simulink model "wlan_mac_dcf_hw"  (Simulink 7.7)
settings: Solver=ode45  StartTime=0.0  StopTime=2e4  RelTol=1e-3
PostLoadFcn:
  | wlan_mac_hw_init
InitFcn:
  | wlan_mac_hw_init
StartFcn:
  | wlan_mac_hw_init
values from neighbouring files (symbols this model uses):
  NB_CNTR_NAV = ceil(log2(MAX_NAV * 160))    [wlan_mac_hw_init.m]
  ticks_per_usec = 10    [wlan_mac_hw_init.m]
undefined symbols (not defined in the file or in its folder): gcbh, xlBlockLoadCallback, xlGetNormalizedPeriod
libraries: xbsIndex_r4 x552, xbsEDKLib_r4 x1
(part 4 of 5)

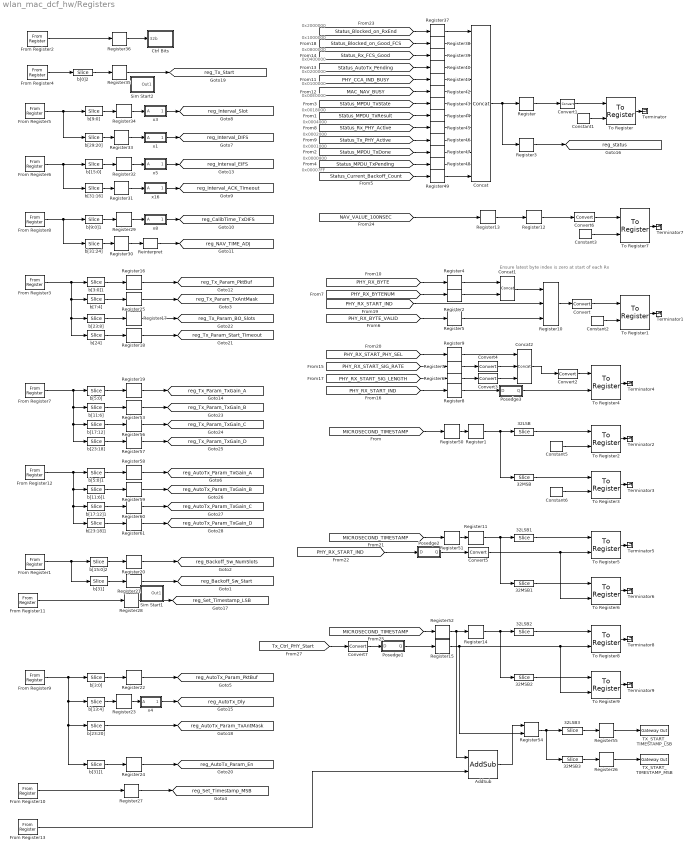
== system wlan_mac_dcf_hw/Registers ==
  note: Ensure latest byte index is zero
      | at start of each Rx
  note: 0x00007FF
  note: 0x0000800
  note: 0x0001000
  note: 0x0002000
  note: 0x0004000
  note: 0x0018000
  note: 0x00E0000
  note: 0x0100000
  note: 0x0200000
  note: 0x0400000
  note: 0x0800000
  note: 0x1000000
  note: 0x2000000
  " b[11:6]" : xbsIndex_r4/Slice  nbits=6  boolean_output=off  mode=Lower Bit Location + Width  bit1=0  base1=MSB of Input  bit0=6  base0=LSB of Input  dbl_ovrd=off  block_type=slice
      settings: block_version=VER_STRING_GOES_HERE
  " b[11:6]1" : xbsIndex_r4/Slice  nbits=6  boolean_output=off  mode=Lower Bit Location + Width  bit1=0  base1=MSB of Input  bit0=6  base0=LSB of Input  dbl_ovrd=off  block_type=slice
      settings: block_version=VER_STRING_GOES_HERE
  " b[13:4]" : xbsIndex_r4/Slice  nbits=10  boolean_output=off  mode=Lower Bit Location + Width  bit1=0  base1=MSB of Input  bit0=4  base0=LSB of Input  dbl_ovrd=off  block_type=slice
      settings: block_version=VER_STRING_GOES_HERE
  " b[15:0]" : xbsIndex_r4/Slice  nbits=16  boolean_output=off  mode=Lower Bit Location + Width  bit1=0  base1=MSB of Input  bit0=0  base0=LSB of Input  dbl_ovrd=off  block_type=slice
      settings: block_version=VER_STRING_GOES_HERE
  " b[15:0]2" : xbsIndex_r4/Slice  nbits=16  boolean_output=off  mode=Lower Bit Location + Width  bit1=0  base1=MSB of Input  bit0=0  base0=LSB of Input  dbl_ovrd=off  block_type=slice
      settings: block_version=VER_STRING_GOES_HERE
  " b[17:12]" : xbsIndex_r4/Slice  nbits=6  boolean_output=off  mode=Lower Bit Location + Width  bit1=0  base1=MSB of Input  bit0=12  base0=LSB of Input  dbl_ovrd=off  block_type=slice
      settings: block_version=VER_STRING_GOES_HERE
  " b[17:12]1" : xbsIndex_r4/Slice  nbits=6  boolean_output=off  mode=Lower Bit Location + Width  bit1=0  base1=MSB of Input  bit0=12  base0=LSB of Input  dbl_ovrd=off  block_type=slice
      settings: block_version=VER_STRING_GOES_HERE
  " b[23:18]" : xbsIndex_r4/Slice  nbits=6  boolean_output=off  mode=Lower Bit Location + Width  bit1=0  base1=MSB of Input  bit0=18  base0=LSB of Input  dbl_ovrd=off  block_type=slice
      settings: block_version=VER_STRING_GOES_HERE
  " b[23:18]1" : xbsIndex_r4/Slice  nbits=6  boolean_output=off  mode=Lower Bit Location + Width  bit1=0  base1=MSB of Input  bit0=18  base0=LSB of Input  dbl_ovrd=off  block_type=slice
      settings: block_version=VER_STRING_GOES_HERE
  " b[23:20]" : xbsIndex_r4/Slice  nbits=4  boolean_output=off  mode=Lower Bit Location + Width  bit1=0  base1=MSB of Input  bit0=20  base0=LSB of Input  dbl_ovrd=off  block_type=slice
      settings: block_version=VER_STRING_GOES_HERE
  " b[23:8]" : xbsIndex_r4/Slice  nbits=16  boolean_output=off  mode=Lower Bit Location + Width  bit1=0  base1=MSB of Input  bit0=8  base0=LSB of Input  dbl_ovrd=off  block_type=slice
      settings: block_version=VER_STRING_GOES_HERE
  " b[24]" : xbsIndex_r4/Slice  nbits=1  boolean_output=on  mode=Lower Bit Location + Width  bit1=0  base1=MSB of Input  bit0=24  base0=LSB of Input  dbl_ovrd=off  block_type=slice
      settings: block_version=VER_STRING_GOES_HERE
  " b[29:20]" : xbsIndex_r4/Slice  nbits=10  boolean_output=off  mode=Lower Bit Location + Width  bit1=0  base1=MSB of Input  bit0=20  base0=LSB of Input  dbl_ovrd=off  block_type=slice
      settings: block_version=VER_STRING_GOES_HERE
  " b[31:16]" : xbsIndex_r4/Slice  nbits=16  boolean_output=off  mode=Lower Bit Location + Width  bit1=0  base1=MSB of Input  bit0=16  base0=LSB of Input  dbl_ovrd=off  block_type=slice
      settings: block_version=VER_STRING_GOES_HERE
  " b[31:24]" : xbsIndex_r4/Slice  nbits=8  boolean_output=off  mode=Lower Bit Location + Width  bit1=0  base1=MSB of Input  bit0=24  base0=LSB of Input  dbl_ovrd=off  block_type=slice
      settings: block_version=VER_STRING_GOES_HERE
  " b[31]" : xbsIndex_r4/Slice  nbits=1  boolean_output=on  mode=Lower Bit Location + Width  bit1=0  base1=MSB of Input  bit0=31  base0=LSB of Input  dbl_ovrd=off  block_type=slice
      settings: block_version=VER_STRING_GOES_HERE
  " b[31]1" : xbsIndex_r4/Slice  nbits=1  boolean_output=on  mode=Lower Bit Location + Width  bit1=0  base1=MSB of Input  bit0=31  base0=LSB of Input  dbl_ovrd=off  block_type=slice
      settings: block_version=VER_STRING_GOES_HERE
  " b[3:0]" : xbsIndex_r4/Slice  nbits=4  boolean_output=off  mode=Lower Bit Location + Width  bit1=0  base1=MSB of Input  bit0=0  base0=LSB of Input  dbl_ovrd=off  block_type=slice
      settings: block_version=VER_STRING_GOES_HERE
  " b[3:0]1" : xbsIndex_r4/Slice  nbits=4  boolean_output=off  mode=Lower Bit Location + Width  bit1=0  base1=MSB of Input  bit0=0  base0=LSB of Input  dbl_ovrd=off  block_type=slice
      settings: block_version=VER_STRING_GOES_HERE
  " b[5:0]" : xbsIndex_r4/Slice  nbits=6  boolean_output=off  mode=Lower Bit Location + Width  bit1=0  base1=MSB of Input  bit0=0  base0=LSB of Input  dbl_ovrd=off  block_type=slice
      settings: block_version=VER_STRING_GOES_HERE
  " b[5:0]1" : xbsIndex_r4/Slice  nbits=6  boolean_output=off  mode=Lower Bit Location + Width  bit1=0  base1=MSB of Input  bit0=0  base0=LSB of Input  dbl_ovrd=off  block_type=slice
      settings: block_version=VER_STRING_GOES_HERE
  " b[7:4]" : xbsIndex_r4/Slice  nbits=4  boolean_output=off  mode=Lower Bit Location + Width  bit1=0  base1=MSB of Input  bit0=4  base0=LSB of Input  dbl_ovrd=off  block_type=slice
      settings: block_version=VER_STRING_GOES_HERE
  " b[9:0]" : xbsIndex_r4/Slice  nbits=10  boolean_output=off  mode=Lower Bit Location + Width  bit1=0  base1=MSB of Input  bit0=0  base0=LSB of Input  dbl_ovrd=off  block_type=slice
      settings: block_version=VER_STRING_GOES_HERE
  " b[9:0]1" : xbsIndex_r4/Slice  nbits=10  boolean_output=off  mode=Lower Bit Location + Width  bit1=0  base1=MSB of Input  bit0=0  base0=LSB of Input  dbl_ovrd=off  block_type=slice
      settings: block_version=VER_STRING_GOES_HERE
  32LSB{,1..3} (4 alike) : xbsIndex_r4/Slice  nbits=32  boolean_output=off  mode=Lower Bit Location + Width  bit1=0  base1=MSB of Input  bit0=0  base0=LSB of Input  dbl_ovrd=off  block_type=slice
      settings: block_version=VER_STRING_GOES_HERE
  32MSB{,1..3} (4 alike) : xbsIndex_r4/Slice  nbits=32  boolean_output=off  mode=Upper Bit Location + Width  bit1=0  base1=MSB of Input  bit0=0  base0=LSB of Input  dbl_ovrd=off  block_type=slice
      settings: block_version=VER_STRING_GOES_HERE
  AddSub : xbsIndex_r4/AddSub  mode=Addition  use_carryin=off  use_carryout=off  en=off  latency=0  precision=User Defined  arith_type=Unsigned  n_bits=64  bin_pt=0  quantization=Truncate  overflow=Wrap  dbl_ovrd=off  use_behavioral_HDL=off  hw_selection=Fabric  pipelined=off  block_type=addsub
  Concat : xbsIndex_r4/Concat  num_inputs=13  dbl_ovrd=off  block_type=concat
      settings: block_version=8.2.02
  Concat1 : xbsIndex_r4/Concat  num_inputs=2  dbl_ovrd=off  block_type=concat
      settings: block_version=8.2.02
  Concat2 : xbsIndex_r4/Concat  num_inputs=3  dbl_ovrd=off  block_type=concat
      settings: block_version=8.2.02
  Constant{1..3,5..6} (5 alike) : xbsIndex_r4/Constant  const=1  gui_display_data_type=Boolean  arith_type=Boolean  n_bits=30  bin_pt=0  preci_type=Single  exp_width=8  frac_width=24  explicit_period=on  period=1  equ=P=C  opselect=C  inp2=PCIN>>17  opr=+  inp1=P  carry=CIN  dbl_ovrd=off  block_type=constant
  Convert{,1..2,6} (4 alike) : xbsIndex_r4/Convert  gui_display_data_type=Fixed-point  arith_type=Unsigned  n_bits=32  bin_pt=0  float_type=Single  exp_bits=8  fraction_bits=24  quantization=Truncate  overflow=Wrap  en=off  latency=0  dbl_ovrd=off  pipeline=off  block_type=convert
  Convert3 : xbsIndex_r4/Convert  gui_display_data_type=Fixed-point  arith_type=Unsigned  n_bits=16  bin_pt=0  float_type=Single  exp_bits=8  fraction_bits=24  quantization=Truncate  overflow=Wrap  en=off  latency=0  dbl_ovrd=off  pipeline=off  block_type=convert
  Convert4 : xbsIndex_r4/Convert  gui_display_data_type=Fixed-point  arith_type=Unsigned  n_bits=8  bin_pt=0  float_type=Single  exp_bits=8  fraction_bits=24  quantization=Truncate  overflow=Wrap  en=off  latency=0  dbl_ovrd=off  pipeline=off  block_type=convert
  Convert5 : xbsIndex_r4/Convert  gui_display_data_type=Boolean  arith_type=Boolean  n_bits=32  bin_pt=0  float_type=Single  exp_bits=8  fraction_bits=24  quantization=Truncate  overflow=Wrap  en=off  latency=0  dbl_ovrd=off  pipeline=off  block_type=convert
  Convert7 : xbsIndex_r4/Convert  gui_display_data_type=Boolean  arith_type=Boolean  n_bits=32  bin_pt=0  float_type=Single  exp_bits=8  fraction_bits=24  quantization=Truncate  overflow=Wrap  en=off  latency=0  dbl_ovrd=off  pipeline=off  block_type=convert
  Ctrl Bits : Subsystem
  From Register1 : xbsIndex_r4/From Register  shared_memory_name='BACKOFF_CTRL'  init=REG_MAC_Backoff_Control  period=1  ownership=Locally owned and initialized  gui_display_data_type=Fixed-point  arith_type=Unsigned  n_bits=32  bin_pt=0  preci_type=Single  dbl_ovrd=off  block_type=fromreg
      settings: AttributesFormatString=<< %<shared_memory_name> >>  infoedit="Register block that reads data to a shared memory register.  Delay of one sample period."
  From Register10 : xbsIndex_r4/From Register  shared_memory_name='TIMESTAMP_SET_MSB'  init=0  period=1  ownership=Locally owned and initialized  gui_display_data_type=Fixed-point  arith_type=Unsigned  n_bits=32  bin_pt=0  preci_type=Single  dbl_ovrd=off  block_type=fromreg
      settings: AttributesFormatString=<< %<shared_memory_name> >>  infoedit="Register block that reads data to a shared memory register.  Delay of one sample period."
  From Register11 : xbsIndex_r4/From Register  shared_memory_name='TIMESTAMP_SET_LSB'  init=0  period=1  ownership=Locally owned and initialized  gui_display_data_type=Fixed-point  arith_type=Unsigned  n_bits=32  bin_pt=0  preci_type=Single  dbl_ovrd=off  block_type=fromreg
      settings: AttributesFormatString=<< %<shared_memory_name> >>  infoedit="Register block that reads data to a shared memory register.  Delay of one sample period."
  From Register12 : xbsIndex_r4/From Register  shared_memory_name='AUTO_TX_GAINS'  init=0  period=1  ownership=Locally owned and initialized  gui_display_data_type=Fixed-point  arith_type=Unsigned  n_bits=32  bin_pt=0  preci_type=Single  dbl_ovrd=off  block_type=fromreg
      settings: AttributesFormatString=<< %<shared_memory_name> >>  infoedit="Register block that reads data to a shared memory register.  Delay of one sample period."
  From Register13 : xbsIndex_r4/From Register  shared_memory_name='TIMESTAMP_INSERT_OFFSET'  init=0  period=1  ownership=Locally owned and initialized  gui_display_data_type=Fixed-point  arith_type="Signed  (2's comp)"  n_bits=32  bin_pt=0  preci_type=Single  dbl_ovrd=off  block_type=fromreg
      settings: AttributesFormatString=<< %<shared_memory_name> >>  infoedit="Register block that reads data to a shared memory register.  Delay of one sample period."
  From Register2 : xbsIndex_r4/From Register  shared_memory_name='Control'  init=REG_MAC_Control  period=1  ownership=Locally owned and initialized  gui_display_data_type=Fixed-point  arith_type=Unsigned  n_bits=32  bin_pt=0  preci_type=Single  dbl_ovrd=off  block_type=fromreg
      settings: AttributesFormatString=<< %<shared_memory_name> >>  infoedit="Register block that reads data to a shared memory register.  Delay of one sample period."
  From Register3 : xbsIndex_r4/From Register  shared_memory_name='MPDU_TX_PARAMS'  init=REG_MAC_MPDU_Tx_Params  period=1  ownership=Locally owned and initialized  gui_display_data_type=Fixed-point  arith_type=Unsigned  n_bits=32  bin_pt=0  preci_type=Single  dbl_ovrd=off  block_type=fromreg
      settings: AttributesFormatString=<< %<shared_memory_name> >>  infoedit="Register block that reads data to a shared memory register.  Delay of one sample period."
  From Register4 : xbsIndex_r4/From Register  shared_memory_name='TX_START'  init=0  period=1  ownership=Locally owned and initialized  gui_display_data_type=Fixed-point  arith_type=Unsigned  n_bits=32  bin_pt=0  preci_type=Single  dbl_ovrd=off  block_type=fromreg
      settings: AttributesFormatString=<< %<shared_memory_name> >>  infoedit="Register block that reads data to a shared memory register.  Delay of one sample period."
  From Register5 : xbsIndex_r4/From Register  shared_memory_name='IFS_INTERVALS1'  init=REG_MAC_Intervals_1  period=1  ownership=Locally owned and initialized  gui_display_data_type=Fixed-point  arith_type=Unsigned  n_bits=32  bin_pt=0  preci_type=Single  dbl_ovrd=off  block_type=fromreg
      settings: AttributesFormatString=<< %<shared_memory_name> >>  infoedit="Register block that reads data to a shared memory register.  Delay of one sample period."
  From Register6 : xbsIndex_r4/From Register  shared_memory_name='IFS_INTERVALS2'  init=REG_MAC_Intervals_2  period=1  ownership=Locally owned and initialized  gui_display_data_type=Fixed-point  arith_type=Unsigned  n_bits=32  bin_pt=0  preci_type=Single  dbl_ovrd=off  block_type=fromreg
      settings: AttributesFormatString=<< %<shared_memory_name> >>  infoedit="Register block that reads data to a shared memory register.  Delay of one sample period."
  From Register7 : xbsIndex_r4/From Register  shared_memory_name='MPDU_TX_GAINS'  init=0  period=1  ownership=Locally owned and initialized  gui_display_data_type=Fixed-point  arith_type=Unsigned  n_bits=32  bin_pt=0  preci_type=Single  dbl_ovrd=off  block_type=fromreg
      settings: AttributesFormatString=<< %<shared_memory_name> >>  infoedit="Register block that reads data to a shared memory register.  Delay of one sample period."
  From Register8 : xbsIndex_r4/From Register  shared_memory_name='CALIB_TIMES'  init=REG_MAC_Calib_Times  period=1  ownership=Locally owned and initialized  gui_display_data_type=Fixed-point  arith_type=Unsigned  n_bits=32  bin_pt=0  preci_type=Single  dbl_ovrd=off  block_type=fromreg
      settings: AttributesFormatString=<< %<shared_memory_name> >>  infoedit="Register block that reads data to a shared memory register.  Delay of one sample period."
  From Register9 : xbsIndex_r4/From Register  shared_memory_name='AUTO_TX_PARAMS'  init=REG_MAC_Auto_Tx_Params  period=1  ownership=Locally owned and initialized  gui_display_data_type=Fixed-point  arith_type=Unsigned  n_bits=32  bin_pt=0  preci_type=Single  dbl_ovrd=off  block_type=fromreg
      settings: AttributesFormatString=<< %<shared_memory_name> >>  infoedit="Register block that reads data to a shared memory register.  Delay of one sample period."
  Posedge1 : Subsystem
  Posedge2 : Subsystem
  Posedge3 : Subsystem
  Register{,1..9,11..53,55..61} (60 alike) : xbsIndex_r4/Register  init=0  rst=off  en=off  dbl_ovrd=off  block_type=register
  Register10 : xbsIndex_r4/Register  init=0  rst=on  en=on  dbl_ovrd=off  block_type=register
  Register54 : xbsIndex_r4/Register  init=0  rst=off  en=on  dbl_ovrd=off  block_type=register
  Reinterpret : xbsIndex_r4/Reinterpret  force_arith_type=on  arith_type="Signed  (2's comp)"  force_bin_pt=off  bin_pt=0  block_type=reinterpret
  Sim Start1 : Subsystem
  Sim Start2 : Subsystem
  TX_START_TIMESTAMP_LSB : xbsIndex_r4/Gateway Out  inherit_from_input=off  hdl_port=on  timing_constraint=None  locs_specified=off  LOCs={}  UseAsDAC=off  DACChannel='1'  block_type=gatewayout
  TX_START_TIMESTAMP_MSB : xbsIndex_r4/Gateway Out  inherit_from_input=off  hdl_port=on  timing_constraint=None  locs_specified=off  LOCs={}  UseAsDAC=off  DACChannel='1'  block_type=gatewayout
  Terminator{,1..9} (10 alike) : Terminator
  To Register : xbsIndex_r4/To Register  shared_memory_name='Status'  init=0  ownership=Locally owned and initialized  explicit_data_type=on  gui_display_data_type=Fixed-point  arith_type=Unsigned  n_bits=32  bin_pt=0  preci_type=Single  dbl_ovrd=off  block_type=toreg
      settings: AttributesFormatString=<< %<shared_memory_name> >>  infoedit="Register block that writes data to a shared memory register.  Delay of one sample period."
  To Register1 : xbsIndex_r4/To Register  shared_memory_name='LATEST_RX_BYTE'  init=0  ownership=Locally owned and initialized  explicit_data_type=on  gui_display_data_type=Fixed-point  arith_type=Unsigned  n_bits=32  bin_pt=0  preci_type=Single  dbl_ovrd=off  block_type=toreg
      settings: AttributesFormatString=<< %<shared_memory_name> >>  infoedit="Register block that writes data to a shared memory register.  Delay of one sample period."
  To Register2 : xbsIndex_r4/To Register  shared_memory_name='TIMESTAMP_LSB'  init=0  ownership=Locally owned and initialized  explicit_data_type=on  gui_display_data_type=Fixed-point  arith_type=Unsigned  n_bits=32  bin_pt=0  preci_type=Single  dbl_ovrd=off  block_type=toreg
      settings: AttributesFormatString=<< %<shared_memory_name> >>  infoedit="Register block that writes data to a shared memory register.  Delay of one sample period."
  To Register3 : xbsIndex_r4/To Register  shared_memory_name='TIMESTAMP_MSB'  init=0  ownership=Locally owned and initialized  explicit_data_type=on  gui_display_data_type=Fixed-point  arith_type=Unsigned  n_bits=32  bin_pt=0  preci_type=Single  dbl_ovrd=off  block_type=toreg
      settings: AttributesFormatString=<< %<shared_memory_name> >>  infoedit="Register block that writes data to a shared memory register.  Delay of one sample period."
  To Register4 : xbsIndex_r4/To Register  shared_memory_name='RX_RATE_LENGTH'  init=0  ownership=Locally owned and initialized  explicit_data_type=on  gui_display_data_type=Fixed-point  arith_type=Unsigned  n_bits=32  bin_pt=0  preci_type=Single  dbl_ovrd=off  block_type=toreg
      settings: AttributesFormatString=<< %<shared_memory_name> >>  infoedit="Register block that writes data to a shared memory register.  Delay of one sample period."
  To Register5 : xbsIndex_r4/To Register  shared_memory_name='RX_START_TIMESTAMP_LSB'  init=0  ownership=Locally owned and initialized  explicit_data_type=on  gui_display_data_type=Fixed-point  arith_type=Unsigned  n_bits=32  bin_pt=0  preci_type=Single  dbl_ovrd=off  block_type=toreg
      settings: AttributesFormatString=<< %<shared_memory_name> >>  infoedit="Register block that writes data to a shared memory register.  Delay of one sample period."
  To Register6 : xbsIndex_r4/To Register  shared_memory_name='RX_START_TIMESTAMP_MSB'  init=0  ownership=Locally owned and initialized  explicit_data_type=on  gui_display_data_type=Fixed-point  arith_type=Unsigned  n_bits=32  bin_pt=0  preci_type=Single  dbl_ovrd=off  block_type=toreg
      settings: AttributesFormatString=<< %<shared_memory_name> >>  infoedit="Register block that writes data to a shared memory register.  Delay of one sample period."
  To Register7 : xbsIndex_r4/To Register  shared_memory_name='NAV_VALUE'  init=0  ownership=Locally owned and initialized  explicit_data_type=on  gui_display_data_type=Fixed-point  arith_type=Unsigned  n_bits=32  bin_pt=0  preci_type=Single  dbl_ovrd=off  block_type=toreg
      settings: AttributesFormatString=<< %<shared_memory_name> >>  infoedit="Register block that writes data to a shared memory register.  Delay of one sample period."
  To Register8 : xbsIndex_r4/To Register  shared_memory_name='TX_START_TIMESTAMP_LSB'  init=0  ownership=Locally owned and initialized  explicit_data_type=on  gui_display_data_type=Fixed-point  arith_type=Unsigned  n_bits=32  bin_pt=0  preci_type=Single  dbl_ovrd=off  block_type=toreg
      settings: AttributesFormatString=<< %<shared_memory_name> >>  infoedit="Register block that writes data to a shared memory register.  Delay of one sample period."
  To Register9 : xbsIndex_r4/To Register  shared_memory_name='TX_START_TIMESTAMP_MSB'  init=0  ownership=Locally owned and initialized  explicit_data_type=on  gui_display_data_type=Fixed-point  arith_type=Unsigned  n_bits=32  bin_pt=0  preci_type=Single  dbl_ovrd=off  block_type=toreg
      settings: AttributesFormatString=<< %<shared_memory_name> >>  infoedit="Register block that writes data to a shared memory register.  Delay of one sample period."
  b[0]2 : xbsIndex_r4/Slice  nbits=1  boolean_output=on  mode=Lower Bit Location + Width  bit1=0  base1=MSB of Input  bit0=0  base0=LSB of Input  dbl_ovrd=off  block_type=slice
      settings: block_version=VER_STRING_GOES_HERE
  x1 : Subsystem
  x16 : Subsystem
  x3 : Subsystem
  x4 : Subsystem
  x5 : Subsystem
  x8 : Subsystem
  tag scope: reg_AutoTx_Dly=global, reg_AutoTx_Param_En=global, reg_AutoTx_Param_PktBuf=global, reg_AutoTx_Param_TxAntMask=global, reg_AutoTx_Param_TxGain_A=global, reg_AutoTx_Param_TxGain_B=global, reg_AutoTx_Param_TxGain_C=global, reg_AutoTx_Param_TxGain_D=global, reg_Backoff_Sw_NumSlots=global, reg_Backoff_Sw_Start=global, reg_CalibTime_TxDIFS=global, reg_Interval_ACK_Timeout=global, reg_Interval_DIFS=global, reg_Interval_EIFS=global, reg_Interval_Slot=global, reg_NAV_TIME_ADJ=global, reg_Set_Timestamp_LSB=global, reg_Set_Timestamp_MSB=global, reg_Tx_Param_BO_Slots=global, reg_Tx_Param_PktBuf=global, reg_Tx_Param_Start_Timeout=global, reg_Tx_Param_TxAntMask=global, reg_Tx_Param_TxGain_A=global, reg_Tx_Param_TxGain_B=global, reg_Tx_Param_TxGain_C=global, reg_Tx_Param_TxGain_D=global, reg_Tx_Start=global, reg_status=global
  wires:
  From Register2/1 -> Register36/1
  Constant1/1 -> To Register/2
  To Register/1 -> Terminator/1
  Concat/1 -> Register3/1, Register/1
  32LSB/1 -> To Register2/1
  Constant5/1 -> To Register2/2
  32MSB/1 -> To Register3/1
  Constant6/1 -> To Register3/2
  [MICROSECOND_TIMESTAMP] -> Register50/1
  x16/1(Ax16) -> [reg_Interval_ACK_Timeout]
  x1/1(Ax16) -> [reg_Interval_DIFS]
  x3/1(Ax16) -> [reg_Interval_Slot]
  x5/1(Ax16) -> [reg_Interval_EIFS]
  From Register3/1 -> " b[3:0]1"/1, " b[23:8]"/1, " b[24]"/1, " b[7:4]"/1
  b[0]2/1 -> Register35/1
  From Register5/1 -> " b[9:0]"/1, " b[29:20]"/1
  From Register6/1 -> " b[15:0]"/1, " b[31:16]"/1
  " b[9:0]"/1 -> Register34/1
  " b[29:20]"/1 -> Register33/1
  " b[15:0]"/1 -> Register32/1
  " b[31:16]"/1 -> Register31/1
  x8/1(Ax16) -> [reg_CalibTime_TxDIFS]
  From Register8/1 -> " b[9:0]1"/1, " b[31:24]"/1
  " b[9:0]1"/1 -> Register29/1
  " b[31:24]"/1 -> Register30/1
  " b[24]"/1 -> Register18/1
  From Register1/1 -> " b[15:0]2"/1, " b[31]"/1
  " b[15:0]2"/1 -> Register20/1
  " b[31]"/1 -> Register21/1
  From Register9/1 -> " b[3:0]"/1, " b[13:4]"/1, " b[23:20]"/1, " b[31]1"/1
  " b[3:0]"/1 -> Register22/1
  To Register1/1 -> Terminator1/1
  [PHY_RX_BYTE_VALID] -> Register5/1
  [PHY_RX_BYTENUM] -> Register2/1
  " b[3:0]1"/1 -> Register16/1
  " b[23:8]"/1 -> Register17/1
  " b[31]1"/1 -> Register24/1
  " b[13:4]"/1 -> Register23/1
  x4/1(Ax16) -> [reg_AutoTx_Dly]
  Register/1 -> Convert1/1
  Register1/1 -> 32LSB/1, 32MSB/1
  Register2/1 -> Concat1/2
  Convert1/1 -> To Register/1
  Register3/1 -> [reg_status]
  Register4/1 -> Concat1/1
  Register5/1 -> Register10/3
  [PHY_RX_BYTE] -> Register4/1
  To Register2/1 -> Terminator2/1
  To Register3/1 -> Terminator3/1
  From Register4/1 -> b[0]2/1
  [PHY_CCA_IND_BUSY] -> Register41/1
  [MAC_NAV_BUSY] -> Register42/1
  [Status_MPDU_TxState] -> Register43/1
  [Status_MPDU_TxResult] -> Register44/1
  [Status_Rx_PHY_Active] -> Register45/1
  [Status_Tx_PHY_Active] -> Register46/1
  [Status_MPDU_TxDone] -> Register47/1
  [Status_MPDU_TxPending] -> Register48/1
  [Status_Current_Backoff_Count] -> Register49/1
  Concat1/1 -> Register10/1
  [Status_AutoTx_Pending] -> Register40/1
  [Status_Rx_FCS_Good] -> Register39/1
  To Register4/1 -> Terminator4/1
  [PHY_RX_START_SIG_LENGTH] -> Register6/1
  Register6/1 -> Convert3/1
  Register7/1 -> Convert4/1
  Register8/1 -> Posedge3/1(D)
  [PHY_RX_START_SIG_RATE] -> Register7/1
  Convert2/1 -> To Register4/1
  [PHY_RX_START_IND] -> Register8/1
  Convert3/1 -> Concat2/3
  [Status_Blocked_on_Good_FCS] -> Register38/1
  [PHY_RX_START_PHY_SEL] -> Register9/1
  Convert4/1 -> Concat2/2
  Register9/1 -> Concat2/1
  Concat2/1 -> Convert2/1
  Register10/1 -> Convert/1
  Convert/1 -> To Register1/1
  Constant2/1 -> To Register1/2
  [PHY_RX_START_IND] -> Register10/2
  32LSB1/1 -> To Register5/1
  [PHY_RX_START_IND] -> Posedge2/1(D)
  32MSB1/1 -> To Register6/1
  [MICROSECOND_TIMESTAMP] -> Register51/1
  Register11/1 -> 32MSB1/1, 32LSB1/1
  To Register5/1 -> Terminator5/1
  To Register6/1 -> Terminator6/1
  Convert5/1 -> To Register5/2, To Register6/2
  From Register11/1 -> Register28/1
  From Register10/1 -> Register27/1
  [Status_Blocked_on_RxEnd] -> Register37/1
  Reinterpret/1 -> [reg_NAV_TIME_ADJ]
  To Register7/1 -> Terminator7/1
  [NAV_VALUE_100NSEC] -> Register13/1
  Convert6/1 -> To Register7/1
  Register12/1 -> Convert6/1
  Register13/1 -> Register12/1
  Constant3/1 -> To Register7/2
  32LSB2/1 -> To Register8/1
  [Tx_Ctrl_PHY_Start] -> Convert7/1
  32MSB2/1 -> To Register9/1
  [MICROSECOND_TIMESTAMP] -> Register52/1
  Register14/1 -> 32LSB2/1, 32MSB2/1
  To Register8/1 -> Terminator8/1
  To Register9/1 -> Terminator9/1
  Register15/1 -> Register54/2, To Register9/2, To Register8/2
  " b[5:0]"/1 -> Register19/1
  Register16/1 -> [reg_Tx_Param_PktBuf]
  Register17/1 -> [reg_Tx_Param_BO_Slots]
  Register18/1 -> [reg_Tx_Param_Start_Timeout]
  Register19/1 -> [reg_Tx_Param_TxGain_A]
  Register20/1 -> [reg_Backoff_Sw_NumSlots]
  Register21/1 -> [reg_Backoff_Sw_Start]
  Register22/1 -> [reg_AutoTx_Param_PktBuf]
  Register23/1 -> x4/1(A)
  Register24/1 -> [reg_AutoTx_Param_En]
  Register27/1 -> [reg_Set_Timestamp_MSB]
  Register28/1 -> [reg_Set_Timestamp_LSB]
  Register29/1 -> x8/1(A)
  Register30/1 -> Reinterpret/1
  Register31/1 -> x16/1(A)
  Register32/1 -> x5/1(A)
  Register33/1 -> x1/1(A)
  Register34/1 -> x3/1(A)
  Register35/1 -> [reg_Tx_Start]
  Register36/1 -> Ctrl Bits/1(32b)
  Register37/1 -> Concat/1
  Register38/1 -> Concat/2
  Register39/1 -> Concat/3
  Register40/1 -> Concat/4
  Register41/1 -> Concat/5
  Register42/1 -> Concat/6
  Register43/1 -> Concat/7
  Register44/1 -> Concat/8
  Register45/1 -> Concat/9
  Register46/1 -> Concat/10
  Register47/1 -> Concat/11
  Register48/1 -> Concat/12
  Register49/1 -> Concat/13
  Register50/1 -> Register1/1
  Register51/1 -> Register11/1
  Register52/1 -> AddSub/1, Register14/1
  Posedge1/1(Q) -> Register15/1
  Posedge2/1(Q) -> Convert5/1
  Posedge3/1(Q) -> To Register4/2
  " b[7:4]"/1 -> Register25/1
  Register25/1 -> [reg_Tx_Param_TxAntMask]
  " b[23:20]"/1 -> [reg_AutoTx_Param_TxAntMask]
  Register26/1 -> TX_START_TIMESTAMP_MSB/1
  Register54/1 -> 32LSB3/1, 32MSB3/1
  Register55/1 -> TX_START_TIMESTAMP_LSB/1
  32LSB3/1 -> Register55/1
  Convert7/1 -> Posedge1/1(D)
  32MSB3/1 -> Register26/1
  From Register7/1 -> " b[5:0]"/1, " b[11:6]"/1, " b[17:12]"/1, " b[23:18]"/1
  " b[11:6]"/1 -> Register53/1
  " b[17:12]"/1 -> Register56/1
  " b[23:18]"/1 -> Register57/1
  Register53/1 -> [reg_Tx_Param_TxGain_B]
  Register56/1 -> [reg_Tx_Param_TxGain_C]
  Register57/1 -> [reg_Tx_Param_TxGain_D]
  " b[5:0]1"/1 -> Register58/1
  Register58/1 -> [reg_AutoTx_Param_TxGain_A]
  From Register12/1 -> " b[5:0]1"/1, " b[11:6]1"/1, " b[17:12]1"/1, " b[23:18]1"/1
  " b[11:6]1"/1 -> Register59/1
  " b[17:12]1"/1 -> Register60/1
  " b[23:18]1"/1 -> Register61/1
  Register59/1 -> [reg_AutoTx_Param_TxGain_B]
  Register60/1 -> [reg_AutoTx_Param_TxGain_C]
  Register61/1 -> [reg_AutoTx_Param_TxGain_D]
  From Register13/1 -> AddSub/2
  AddSub/1 -> Register54/1

== system wlan_mac_dcf_hw/Resets ==
  Convert1 : xbsIndex_r4/Convert  gui_display_data_type=Boolean  arith_type=Boolean  n_bits=16  bin_pt=14  float_type=Single  exp_bits=8  fraction_bits=24  quantization=Truncate  overflow=Wrap  en=off  latency=0  dbl_ovrd=off  pipeline=off  block_type=convert
  tag scope: GLOBAL_RESET=global
  wires:
  [reg_Global_Reset] -> Convert1/1
  Convert1/1 -> [GLOBAL_RESET]

== system wlan_mac_dcf_hw/Timeout ==
  Inverter : xbsIndex_r4/Inverter  en=off  latency=0  dbl_ovrd=off  block_type=inv
      settings: xl_area=[0 0 0 0 0 0 0]  block_version=VER_STRING_GOES_HERE
  Logical2 : xbsIndex_r4/Logical  logical_function=OR  inputs=2  en=off  latency=0  precision=Full  arith_type=Unsigned  n_bits=8  bin_pt=2  align_bp=on  dbl_ovrd=off  block_type=logical
      settings: xl_area=[1 0 0 1 0 0 0]  block_version=VER_STRING_GOES_HERE
  Logical3 : xbsIndex_r4/Logical  logical_function=OR  inputs=3  en=off  latency=0  precision=Full  arith_type=Unsigned  n_bits=8  bin_pt=2  align_bp=on  dbl_ovrd=off  block_type=logical
      settings: xl_area=[1 0 0 1 0 0 0]  block_version=VER_STRING_GOES_HERE
  Posedge1 : Subsystem
  Posedge2 : Subsystem
  Relational2 : xbsIndex_r4/Relational  mode=a>=b  en=off  latency=0  dbl_ovrd=off  block_type=relational
  S-R Latch1 : Subsystem
  Timeout Counter : xbsIndex_r4/Counter  cnt_type=Free Running  cnt_to=Inf  operation=Up  start_count=1  cnt_by_val=1  arith_type=Unsigned  n_bits=NB_CNTR_ACKTIMEOUT  bin_pt=0  load_pin=off  rst=on  en=on  explicit_period=off  period=1  dbl_ovrd=off  use_behavioral_HDL=off  implementation=Fabric  block_type=counter
  Timeout Done : Outport
  wires:
  Posedge1/1(Q) -> Timeout Done/1
  Posedge2/1(Q) -> S-R Latch1/1(S)
  [Tx_Ctrl_Timeout_Start] -> Posedge2/1(D)
  Timeout Counter/1 -> Relational2/1
  [reg_Interval_ACK_Timeout] -> Relational2/2
  Relational2/1 -> Posedge1/1(D), Logical2/1, Logical3/3
  Logical2/1 -> Timeout Counter/1
  Inverter/1 -> Logical2/2
  [PHY_RX_START_IND] -> Logical3/1
  Logical3/1 -> S-R Latch1/2(R)
  [GLOBAL_RESET] -> Logical3/2
  S-R Latch1/1(Q) -> Timeout Counter/2, Inverter/1

== system wlan_mac_dcf_hw/64-bit usec  Counter/Posedge2 ==
  note: Rising Edge Detection
  D : Inport
  Delay : xbsIndex_r4/Delay  rst=off  infoeditControl=Selection of Reset will increase slice count due to use of real FFs and instead of SRLs  en=off  latency=1  dbl_ovrd=off  reg_retiming=off  block_type=delay
      settings: infoedit=Hardware notes: A delay line is a chain, each link of which is an SRL16 followed by a flip-flop. If register retiming is enabled, the delay line is a chain of flip-flops.  xl_area=[1 1 0 0 0 0 0]  block_version=VER_STRING_GOES_HERE
  Inverter : xbsIndex_r4/Inverter  en=off  latency=0  dbl_ovrd=off  block_type=inv
      settings: xl_area=[0 0 0 0 0 0 0]  block_version=VER_STRING_GOES_HERE
  Logical1 : xbsIndex_r4/Logical  logical_function=AND  inputs=2  en=off  latency=0  precision=Full  arith_type=Unsigned  n_bits=8  bin_pt=2  align_bp=on  dbl_ovrd=off  block_type=logical
      settings: xl_area=[1 0 0 1 0 0 0]  block_version=VER_STRING_GOES_HERE
  Q : Outport
  wires:
  D/1 -> Logical1/2, Delay/1
  Logical1/1 -> Q/1
  Inverter/1 -> Logical1/1
  Delay/1 -> Inverter/1

== system wlan_mac_dcf_hw/64-bit usec  Counter/usec Pulse ==
  Rst : Inport
  Clk->usec : xbsIndex_r4/Counter  cnt_type=Free Running  cnt_to=159  operation=Up  start_count=0  cnt_by_val=1  arith_type=Unsigned  n_bits=8  bin_pt=0  load_pin=off  rst=on  en=off  explicit_period=off  period=1  dbl_ovrd=off  use_behavioral_HDL=off  implementation=Fabric  block_type=counter
  Constant1 : xbsIndex_r4/Constant  const=159  gui_display_data_type=Fixed-point  arith_type=Unsigned  n_bits=8  bin_pt=0  preci_type=Single  exp_width=8  frac_width=24  explicit_period=off  period=1  equ=P=C  opselect=C  inp2=PCIN>>17  opr=+  inp1=P  carry=CIN  dbl_ovrd=off  block_type=constant
      settings: block_version=8.2.02
  Logical : xbsIndex_r4/Logical  logical_function=OR  inputs=2  en=off  latency=0  precision=Full  arith_type=Unsigned  n_bits=16  bin_pt=0  align_bp=on  dbl_ovrd=off  block_type=logical
  Relational : xbsIndex_r4/Relational  mode=a=b  en=off  latency=0  dbl_ovrd=off  block_type=relational
  uSec : Outport
  wires:
  Clk->usec/1 -> Relational/1
  Constant1/1 -> Relational/2
  Relational/1 -> uSec/1, Logical/1
  Logical/1 -> Clk->usec/1
  Rst/1 -> Logical/2

== system wlan_mac_dcf_hw/Auto Tx Control/Posedge1 ==
  note: Rising Edge Detection
  D : Inport
  Delay : xbsIndex_r4/Delay  rst=off  infoeditControl=Selection of Reset will increase slice count due to use of real FFs and instead of SRLs  en=off  latency=1  dbl_ovrd=off  reg_retiming=off  block_type=delay
      settings: infoedit=Hardware notes: A delay line is a chain, each link of which is an SRL16 followed by a flip-flop. If register retiming is enabled, the delay line is a chain of flip-flops.  xl_area=[1 1 0 0 0 0 0]  block_version=VER_STRING_GOES_HERE
  Inverter : xbsIndex_r4/Inverter  en=off  latency=0  dbl_ovrd=off  block_type=inv
      settings: xl_area=[0 0 0 0 0 0 0]  block_version=VER_STRING_GOES_HERE
  Logical1 : xbsIndex_r4/Logical  logical_function=AND  inputs=2  en=off  latency=0  precision=Full  arith_type=Unsigned  n_bits=8  bin_pt=2  align_bp=on  dbl_ovrd=off  block_type=logical
      settings: xl_area=[1 0 0 1 0 0 0]  block_version=VER_STRING_GOES_HERE
  Q : Outport
  wires:
  Delay/1 -> Inverter/1
  Inverter/1 -> Logical1/1
  Logical1/1 -> Q/1
  D/1 -> Delay/1, Logical1/2

== system wlan_mac_dcf_hw/Auto Tx Control/Posedge2 ==
  note: Rising Edge Detection
  D : Inport
  Delay : xbsIndex_r4/Delay  rst=off  infoeditControl=Selection of Reset will increase slice count due to use of real FFs and instead of SRLs  en=off  latency=1  dbl_ovrd=off  reg_retiming=off  block_type=delay
      settings: infoedit=Hardware notes: A delay line is a chain, each link of which is an SRL16 followed by a flip-flop. If register retiming is enabled, the delay line is a chain of flip-flops.  xl_area=[1 1 0 0 0 0 0]  block_version=VER_STRING_GOES_HERE
  Inverter : xbsIndex_r4/Inverter  en=off  latency=0  dbl_ovrd=off  block_type=inv
      settings: xl_area=[0 0 0 0 0 0 0]  block_version=VER_STRING_GOES_HERE
  Logical1 : xbsIndex_r4/Logical  logical_function=AND  inputs=2  en=off  latency=0  precision=Full  arith_type=Unsigned  n_bits=8  bin_pt=2  align_bp=on  dbl_ovrd=off  block_type=logical
      settings: xl_area=[1 0 0 1 0 0 0]  block_version=VER_STRING_GOES_HERE
  Q : Outport
  wires:
  D/1 -> Logical1/2, Delay/1
  Logical1/1 -> Q/1
  Inverter/1 -> Logical1/1
  Delay/1 -> Inverter/1

== system wlan_mac_dcf_hw/Auto Tx Control/S-R Latch1 ==
  S : Inport
  R : Inport  Port=2
  Constant1 : xbsIndex_r4/Constant  const=1  gui_display_data_type=Boolean  arith_type=Boolean  n_bits=1  bin_pt=0  preci_type=Single  exp_width=8  frac_width=24  explicit_period=off  period=1  equ=P=C  opselect=C  inp2=PCIN>>17  opr=+  inp1=P  carry=CIN  dbl_ovrd=off  block_type=constant
      settings: block_version=VER_STRING_GOES_HERE
  Register2 : xbsIndex_r4/Register  init=0  rst=on  en=on  dbl_ovrd=off  block_type=register
      settings: xl_area=[1 1 0 0 0 0 0]  block_version=VER_STRING_GOES_HERE
  Q : Outport
  wires:
  S/1 -> Register2/3
  Register2/1 -> Q/1
  R/1 -> Register2/2
  Constant1/1 -> Register2/1

== system wlan_mac_dcf_hw/Auto Tx Control/S-R Latch2 ==
  S : Inport
  R : Inport  Port=2
  Constant1 : xbsIndex_r4/Constant  const=1  gui_display_data_type=Boolean  arith_type=Boolean  n_bits=1  bin_pt=0  preci_type=Single  exp_width=8  frac_width=24  explicit_period=off  period=1  equ=P=C  opselect=C  inp2=PCIN>>17  opr=+  inp1=P  carry=CIN  dbl_ovrd=off  block_type=constant
      settings: block_version=VER_STRING_GOES_HERE
  Register2 : xbsIndex_r4/Register  init=0  rst=on  en=on  dbl_ovrd=off  block_type=register
      settings: xl_area=[1 1 0 0 0 0 0]  block_version=VER_STRING_GOES_HERE
  Q : Outport
  wires:
  Constant1/1 -> Register2/1
  R/1 -> Register2/2
  Register2/1 -> Q/1
  S/1 -> Register2/3

== system wlan_mac_dcf_hw/Auto Tx Control/negedge ==
  D : Inport
  Delay : xbsIndex_r4/Delay  rst=off  infoeditControl=Selection of Reset will increase slice count due to use of real FFs and instead of SRLs  en=off  latency=1  dbl_ovrd=off  reg_retiming=off  block_type=delay
      settings: infoedit=Hardware notes: A delay line is a chain, each link of which is an SRL16 followed by a flip-flop. If register retiming is enabled, the delay line is a chain of flip-flops.  xl_area=[1 1 0 0 0 0 0]  block_version=VER_STRING_GOES_HERE
  Inverter : xbsIndex_r4/Inverter  en=off  latency=0  dbl_ovrd=off  block_type=inv
      settings: xl_area=[0 0 0 0 0 0 0]  block_version=VER_STRING_GOES_HERE
  Logical1 : xbsIndex_r4/Logical  logical_function=AND  inputs=2  en=off  latency=0  precision=Full  arith_type=Unsigned  n_bits=8  bin_pt=2  align_bp=on  dbl_ovrd=off  block_type=logical
      settings: xl_area=[1 0 0 1 0 0 0]  block_version=VER_STRING_GOES_HERE
  Q : Outport
  wires:
  Delay/1 -> Logical1/1
  Logical1/1 -> Q/1
  D/1 -> Delay/1, Inverter/1
  Inverter/1 -> Logical1/2

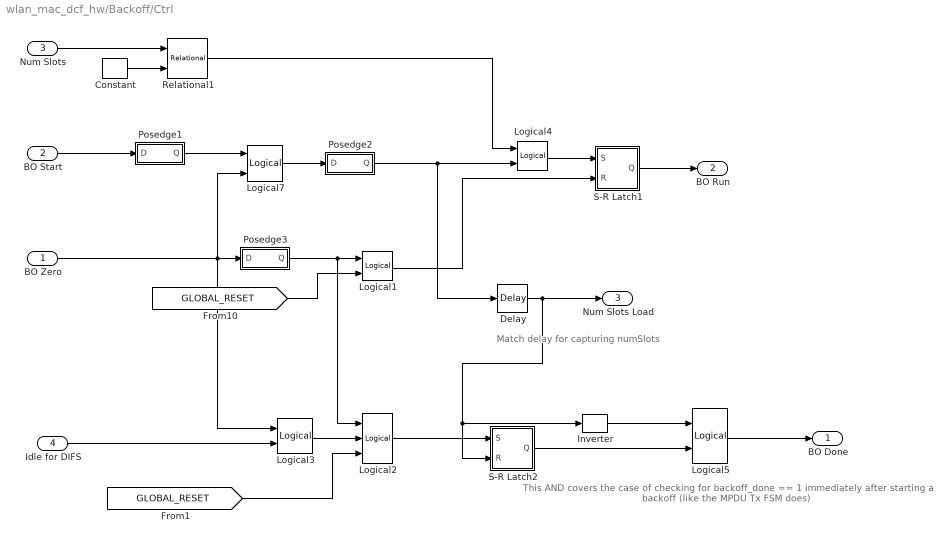
== system wlan_mac_dcf_hw/Backoff/Ctrl ==
  note: Match delay for capturing numSlots
  note: This AND covers the case of checking for
      | backoff_done == 1 immediately after
      | starting a backoff (like the MPDU Tx FSM does)
  BO Zero : Inport
  BO Start : Inport  Port=2
  Num Slots : Inport  Port=3
  Idle for DIFS : Inport  Port=4
  Constant : xbsIndex_r4/Constant  const=0  gui_display_data_type=Fixed-point  arith_type=Unsigned  n_bits=1  bin_pt=0  preci_type=Single  exp_width=8  frac_width=24  explicit_period=off  period=1  equ=P=C  opselect=C  inp2=PCIN>>17  opr=+  inp1=P  carry=CIN  dbl_ovrd=off  block_type=constant
  Delay : xbsIndex_r4/Delay  rst=off  infoeditControl=Selection of Reset will increase slice count due to use of real FFs and instead of SRLs  en=off  latency=1  dbl_ovrd=off  reg_retiming=off  block_type=delay
  Inverter : xbsIndex_r4/Inverter  en=off  latency=0  dbl_ovrd=off  block_type=inv
      settings: xl_area=[0 0 0 0 0 0 0]  block_version=VER_STRING_GOES_HERE
  Logical1 : xbsIndex_r4/Logical  logical_function=OR  inputs=2  en=off  latency=0  precision=Full  arith_type=Unsigned  n_bits=8  bin_pt=2  align_bp=on  dbl_ovrd=off  block_type=logical
      settings: xl_area=[1 0 0 1 0 0 0]  block_version=VER_STRING_GOES_HERE
  Logical2 : xbsIndex_r4/Logical  logical_function=OR  inputs=3  en=off  latency=0  precision=Full  arith_type=Unsigned  n_bits=8  bin_pt=2  align_bp=on  dbl_ovrd=off  block_type=logical
      settings: xl_area=[1 0 0 1 0 0 0]  block_version=VER_STRING_GOES_HERE
  Logical3 : xbsIndex_r4/Logical  logical_function=AND  inputs=2  en=off  latency=0  precision=Full  arith_type=Unsigned  n_bits=16  bin_pt=0  align_bp=on  dbl_ovrd=off  block_type=logical
  Logical4 : xbsIndex_r4/Logical  logical_function=AND  inputs=2  en=off  latency=0  precision=Full  arith_type=Unsigned  n_bits=8  bin_pt=2  align_bp=on  dbl_ovrd=off  block_type=logical
      settings: xl_area=[1 0 0 1 0 0 0]  block_version=VER_STRING_GOES_HERE
  Logical5 : xbsIndex_r4/Logical  logical_function=AND  inputs=2  en=off  latency=0  precision=Full  arith_type=Unsigned  n_bits=16  bin_pt=0  align_bp=on  dbl_ovrd=off  block_type=logical
  Logical7 : xbsIndex_r4/Logical  logical_function=AND  inputs=2  en=off  latency=0  precision=Full  arith_type=Unsigned  n_bits=16  bin_pt=0  align_bp=on  dbl_ovrd=off  block_type=logical
  Posedge1 : Subsystem
  Posedge2 : Subsystem
  Posedge3 : Subsystem
  Relational1 : xbsIndex_r4/Relational  mode=a>b  en=off  latency=0  dbl_ovrd=off  block_type=relational
  S-R Latch1 : Subsystem
  S-R Latch2 : Subsystem
  BO Done : Outport
  BO Run : Outport  Port=2
  Num Slots Load : Outport  Port=3
  wires:
  Logical7/1 -> Posedge2/1(D)
  BO Start/1 -> Posedge1/1(D)
  S-R Latch1/1(Q) -> BO Run/1
  BO Zero/1 -> Logical3/1, Posedge3/1(D), Logical7/2
  Posedge2/1(Q) -> Logical4/2, Delay/1
  Logical1/1 -> S-R Latch1/2(R)
  [GLOBAL_RESET] -> Logical1/2
  Idle for DIFS/1 -> Logical3/2
  [GLOBAL_RESET] -> Logical2/3
  Logical2/1 -> S-R Latch2/1(S)
  Logical3/1 -> Logical2/2
  Posedge3/1(Q) -> Logical2/1, Logical1/1
  Num Slots/1 -> Relational1/1
  Constant/1 -> Relational1/2
  Posedge1/1(Q) -> Logical7/1
  Logical4/1 -> S-R Latch1/1(S)
  Relational1/1 -> Logical4/1
  Delay/1 -> Num Slots Load/1, S-R Latch2/2(R), Inverter/1
  Logical5/1 -> BO Done/1
  S-R Latch2/1(Q) -> Logical5/2
  Inverter/1 -> Logical5/1

== system wlan_mac_dcf_hw/Backoff/Slot Time ==
  note: Counter starts over if it is disabled
  En : Inport
  Gateway Out : xbsIndex_r4/Gateway Out  inherit_from_input=off  hdl_port=off  timing_constraint=None  locs_specified=off  LOCs={}  UseAsDAC=off  DACChannel='1'  block_type=gatewayout
  Gateway Out1 : xbsIndex_r4/Gateway Out  inherit_from_input=off  hdl_port=off  timing_constraint=None  locs_specified=off  LOCs={}  UseAsDAC=off  DACChannel='1'  block_type=gatewayout
  Gateway Out3 : xbsIndex_r4/Gateway Out  inherit_from_input=off  hdl_port=off  timing_constraint=None  locs_specified=off  LOCs={}  UseAsDAC=off  DACChannel='1'  block_type=gatewayout
  Inverter : xbsIndex_r4/Inverter  en=off  latency=0  dbl_ovrd=off  block_type=inv
      settings: xl_area=[0 0 0 0 0 0 0]  block_version=VER_STRING_GOES_HERE
  Logical1 : xbsIndex_r4/Logical  logical_function=OR  inputs=2  en=off  latency=0  precision=Full  arith_type=Unsigned  n_bits=16  bin_pt=0  align_bp=on  dbl_ovrd=off  block_type=logical
  Posedge2 : Subsystem
  Relational2 : xbsIndex_r4/Relational  mode=a>=b  en=off  latency=0  dbl_ovrd=off  block_type=relational
  Slot Time : xbsIndex_r4/Counter  cnt_type=Free Running  cnt_to=Inf  operation=Up  start_count=1  cnt_by_val=1  arith_type=Unsigned  n_bits=NB_CNTR_SLOT  bin_pt=0  load_pin=off  rst=on  en=on  explicit_period=off  period=1  dbl_ovrd=off  use_behavioral_HDL=off  implementation=Fabric  block_type=counter
  Slot Timer : Scope  NumInputPorts=7
      settings: YMin=-5~-5~-5~-5~-5~-5~-5  YMax=5~5~5~5~5~5~5  SaveName=ScopeData5
  Slot Done : Outport
  wires:
  En/1 -> Inverter/1, Slot Time/2, Gateway Out/1
  Inverter/1 -> Logical1/2
  Relational2/1 -> Logical1/1, Posedge2/1(D)
  Logical1/1 -> Slot Time/1
  [reg_Interval_Slot] -> Relational2/2
  Slot Time/1 -> Relational2/1, Gateway Out1/1
  Gateway Out/1 -> Slot Timer/1
  Gateway Out1/1 -> Slot Timer/2
  Gateway Out3/1 -> Slot Timer/4
  Posedge2/1(Q) -> Slot Done/1, Gateway Out3/1

== system wlan_mac_dcf_hw/Idle for DIFS-EIFS/Bad Rx ==
  note: Reception with Errors
  Constant1 : xbsIndex_r4/Constant  const=0  gui_display_data_type=Fixed-point  arith_type=Unsigned  n_bits=1  bin_pt=0  preci_type=Single  exp_width=8  frac_width=24  explicit_period=off  period=1  equ=P=C  opselect=C  inp2=PCIN>>17  opr=+  inp1=P  carry=CIN  dbl_ovrd=off  block_type=constant
  Inverter1 : xbsIndex_r4/Inverter  en=off  latency=0  dbl_ovrd=off  block_type=inv
      settings: xl_area=[0 0 0 0 0 0 0]  block_version=VER_STRING_GOES_HERE
  Logical3 : xbsIndex_r4/Logical  logical_function=AND  inputs=2  en=off  latency=0  precision=Full  arith_type=Unsigned  n_bits=16  bin_pt=0  align_bp=on  dbl_ovrd=off  block_type=logical
  Logical4 : xbsIndex_r4/Logical  logical_function=OR  inputs=2  en=off  latency=0  precision=Full  arith_type=Unsigned  n_bits=16  bin_pt=0  align_bp=on  dbl_ovrd=off  block_type=logical
  Posedge1 : Subsystem
  Relational1 : xbsIndex_r4/Relational  mode=a!=b  en=off  latency=0  dbl_ovrd=off  block_type=relational
  Rx : Outport
  wires:
  [PHY_RX_END_IND] -> Logical3/1
  [PHY_RX_FCS_GOOD_IND] -> Inverter1/1
  Inverter1/1 -> Logical4/1
  Logical4/1 -> Logical3/2
  Constant1/1 -> Relational1/2
  [PHY_RX_END_RXERROR] -> Relational1/1
  Relational1/1 -> Logical4/2
  Logical3/1 -> Posedge1/1(D)
  Posedge1/1(Q) -> Rx/1

== system wlan_mac_dcf_hw/Idle for DIFS-EIFS/S-R Latch1 ==
  S : Inport
  R : Inport  Port=2
  Constant1 : xbsIndex_r4/Constant  const=1  gui_display_data_type=Boolean  arith_type=Boolean  n_bits=1  bin_pt=0  preci_type=Single  exp_width=8  frac_width=24  explicit_period=off  period=1  equ=P=C  opselect=C  inp2=PCIN>>17  opr=+  inp1=P  carry=CIN  dbl_ovrd=off  block_type=constant
      settings: block_version=VER_STRING_GOES_HERE
  Register2 : xbsIndex_r4/Register  init=0  rst=on  en=on  dbl_ovrd=off  block_type=register
      settings: xl_area=[1 1 0 0 0 0 0]  block_version=VER_STRING_GOES_HERE
  Q : Outport
  wires:
  S/1 -> Register2/3
  Register2/1 -> Q/1
  R/1 -> Register2/2
  Constant1/1 -> Register2/1

== system wlan_mac_dcf_hw/MPDU Tx Control/Posedge1 ==
  note: Rising Edge Detection
  D : Inport
  Delay : xbsIndex_r4/Delay  rst=off  infoeditControl=Selection of Reset will increase slice count due to use of real FFs and instead of SRLs  en=off  latency=1  dbl_ovrd=off  reg_retiming=off  block_type=delay
      settings: infoedit=Hardware notes: A delay line is a chain, each link of which is an SRL16 followed by a flip-flop. If register retiming is enabled, the delay line is a chain of flip-flops.  xl_area=[1 1 0 0 0 0 0]  block_version=VER_STRING_GOES_HERE
  Inverter : xbsIndex_r4/Inverter  en=off  latency=0  dbl_ovrd=off  block_type=inv
      settings: xl_area=[0 0 0 0 0 0 0]  block_version=VER_STRING_GOES_HERE
  Logical1 : xbsIndex_r4/Logical  logical_function=AND  inputs=2  en=off  latency=0  precision=Full  arith_type=Unsigned  n_bits=8  bin_pt=2  align_bp=on  dbl_ovrd=off  block_type=logical
      settings: xl_area=[1 0 0 1 0 0 0]  block_version=VER_STRING_GOES_HERE
  Q : Outport
  wires:
  Delay/1 -> Inverter/1
  Inverter/1 -> Logical1/1
  Logical1/1 -> Q/1
  D/1 -> Delay/1, Logical1/2

== system wlan_mac_dcf_hw/MPDU Tx Control/Posedge2 ==
  note: Rising Edge Detection
  D : Inport
  Delay : xbsIndex_r4/Delay  rst=off  infoeditControl=Selection of Reset will increase slice count due to use of real FFs and instead of SRLs  en=off  latency=1  dbl_ovrd=off  reg_retiming=off  block_type=delay
      settings: infoedit=Hardware notes: A delay line is a chain, each link of which is an SRL16 followed by a flip-flop. If register retiming is enabled, the delay line is a chain of flip-flops.  xl_area=[1 1 0 0 0 0 0]  block_version=VER_STRING_GOES_HERE
  Inverter : xbsIndex_r4/Inverter  en=off  latency=0  dbl_ovrd=off  block_type=inv
      settings: xl_area=[0 0 0 0 0 0 0]  block_version=VER_STRING_GOES_HERE
  Logical1 : xbsIndex_r4/Logical  logical_function=AND  inputs=2  en=off  latency=0  precision=Full  arith_type=Unsigned  n_bits=8  bin_pt=2  align_bp=on  dbl_ovrd=off  block_type=logical
      settings: xl_area=[1 0 0 1 0 0 0]  block_version=VER_STRING_GOES_HERE
  Q : Outport
  wires:
  D/1 -> Logical1/2, Delay/1
  Logical1/1 -> Q/1
  Inverter/1 -> Logical1/1
  Delay/1 -> Inverter/1

== system wlan_mac_dcf_hw/MPDU Tx Control/S-R Latch1 ==
  S : Inport
  R : Inport  Port=2
  Constant1 : xbsIndex_r4/Constant  const=1  gui_display_data_type=Boolean  arith_type=Boolean  n_bits=1  bin_pt=0  preci_type=Single  exp_width=8  frac_width=24  explicit_period=off  period=1  equ=P=C  opselect=C  inp2=PCIN>>17  opr=+  inp1=P  carry=CIN  dbl_ovrd=off  block_type=constant
      settings: block_version=VER_STRING_GOES_HERE
  Register2 : xbsIndex_r4/Register  init=0  rst=on  en=on  dbl_ovrd=off  block_type=register
      settings: xl_area=[1 1 0 0 0 0 0]  block_version=VER_STRING_GOES_HERE
  Q : Outport
  wires:
  S/1 -> Register2/3
  Register2/1 -> Q/1
  R/1 -> Register2/2
  Constant1/1 -> Register2/1

== system wlan_mac_dcf_hw/MPDU Tx Control/S-R Latch2 ==
  S : Inport
  R : Inport  Port=2
  Constant1 : xbsIndex_r4/Constant  const=1  gui_display_data_type=Boolean  arith_type=Boolean  n_bits=1  bin_pt=0  preci_type=Single  exp_width=8  frac_width=24  explicit_period=off  period=1  equ=P=C  opselect=C  inp2=PCIN>>17  opr=+  inp1=P  carry=CIN  dbl_ovrd=off  block_type=constant
      settings: block_version=VER_STRING_GOES_HERE
  Register2 : xbsIndex_r4/Register  init=0  rst=on  en=on  dbl_ovrd=off  block_type=register
      settings: xl_area=[1 1 0 0 0 0 0]  block_version=VER_STRING_GOES_HERE
  Q : Outport
  wires:
  Constant1/1 -> Register2/1
  R/1 -> Register2/2
  Register2/1 -> Q/1
  S/1 -> Register2/3
